simulink model "Deployment_Env"  (R2024a)
settings: Solver=ode1  StartTime=0.0  StopTime=inf  FixedStep=0.002  RelTol=1e-3  EnableMultiTasking=on
PostLoadFcn:
  | qc_set_target_type(getConfigSet(bdroot, 'QUARC Default Target Configuration'));
undefined symbols (not defined in the file or in its folder): HIL, Lp, qc_get_step_size
libraries: quarc_library x9, simulink x3, simulink_extras x2, rllib x1
settings Model: SimulationMode=external  ExtModeTrigDuration=5000  Creator=pmartin  LastModifiedBy=sameb
settings SolverCC: AlgebraicLoopSolver=TrustRegion  PositivePriorityOrder=on  AutoInsertRateTranBlk=on
settings DataIOCC: LimitDataPoints=on  SaveFormat=Array  SignalLoggingSaveFormat=ModelDataLogs  ReturnWorkspaceOutputs=off
settings OptimizationCC: ExpressionDepthLimit=2147483647  InitFltsAndDblsToZero=on
settings DebuggingCC: SaveWithParameterizedLinksMsg=none  UnderspecifiedInitializationDetection=Classic  MergeDetectMultiDrivingBlocksExec=none  SolverPrmCheckMsg=warning  MultiTaskDSMMsg=warning  MultiTaskCondExecSysMsg=none  FcnCallInpInsideContextMsg=warning  UnconnectedInputMsg=warning  UnconnectedOutputMsg=warning  UnconnectedLineMsg=warning  StateNameClashWarn=warning  SFUnexpectedBacktrackingDiag=warning  SFNoUnconditionalDefaultTransitionDiag=warning  SFExecutionAtInitializationDiag=none  ArithmeticOperatorsInVariantConditions=warning
settings HardwareCC: ProdBitPerPointer=32  ProdBitPerSizeT=32  ProdBitPerPtrDiffT=32  ProdLargestAtomicFloat=None  ProdIntDivRoundTo=Undefined  ProdEndianess=Unspecified  ProdWordSize=32  ProdHWDeviceType=32-bit Generic
settings ModelReferenceCC: EnableRefExpFcnMdlSchedulingChecks=on  PropagateSignalLabelsOutOfModel=off
settings SFSimCC: SimUseLocalCustomCode=off  CustomCodeUndefinedFunction=UseInterfaceOnly
settings RTWCC: Description=QUARC Win64 Target  SystemTargetFile=quarc_win64.tlc  TemplateMakefile=quarc_default_tmf  RTWUseLocalCustomCode=off  GPUComputeCapability=3.5  DLArmComputeVersion=19.05
settings CodeAppCC: StateflowObjectComments=on
settings STFCustomTargetCC: TargetPreCompLibLocation=C:\PROGRA~3\QUARC\lib\2020b\win64\release  TargetLangStandard=C89/C90 (ANSI)  ConcurrentExecutionCompliant=on  UseToolchainInfoCompliant=off  SystemTargetFile=quarc_win64.tlc
settings GRTTargetCC: TargetPreCompLibLocation=C:\PROGRA~3\QUARC\lib\2020b\win64\release  TargetLangStandard=C89/C90 (ANSI)  ParMdlRefBuildCompliant=off  CompOptLevelCompliant=off  CombineOutputUpdateFcns=off  MatFileLogging=off  CPPClassGenCompliant=off  GRTInterface=on  UseToolchainInfoCompliant=off  ExtMode=on  ExtModeMexFile=quarc_comm
settings ConfigComp: CovMetricSettings=dw  CovSaveCumulativeToWorkspaceVar=on  CovSaveSingleToWorkspaceVar=on  CovExternalEMLEnable=off

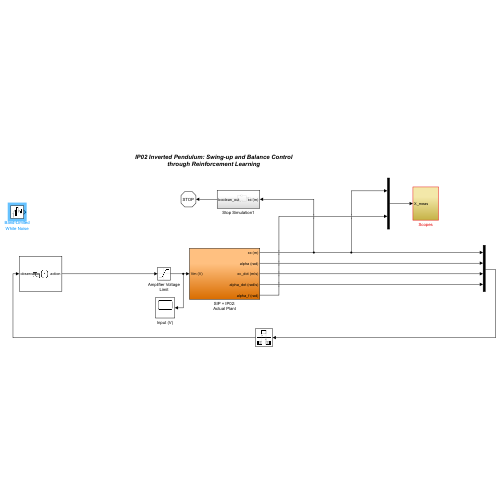
[thumbnail: Simulink's stored preview of the top-level diagram]
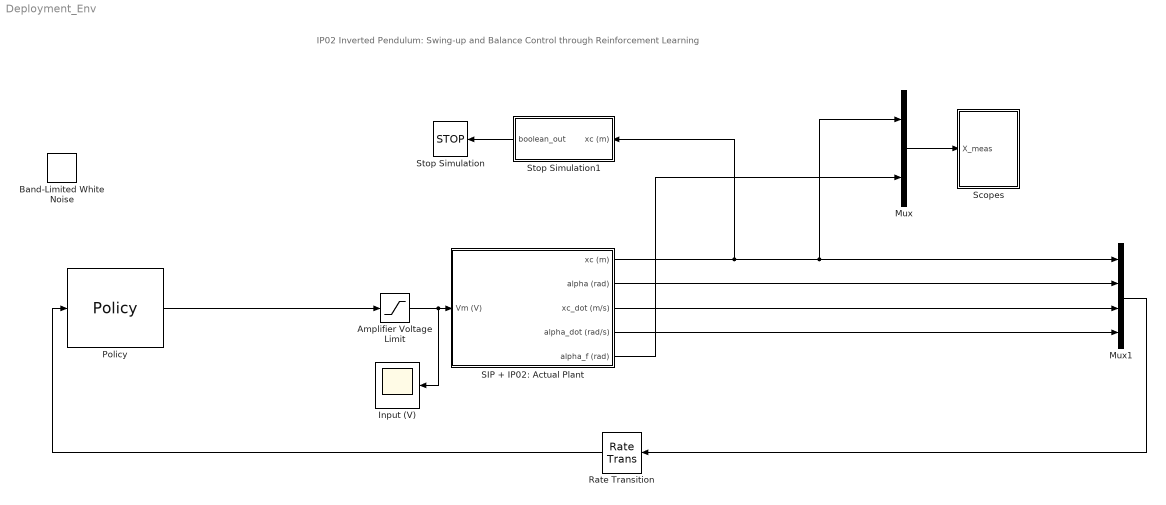
== system Deployment_Env ==
  note: IP02 Inverted Pendulum: Swing-up and Balance Control through Reinforcement Learning
  Amplifier Voltage Limit : Saturate  UpperLimit=10  LowerLimit=-10
  Band-Limited White Noise : simulink/Sources/Band-Limited White Noise  Cov=[0.1]  Ts=0.1  seed=[23341]
  Input (V) : Scope
  Mux : Mux  Inputs=2
  Mux1 : Mux
  Policy : rllib/Policy  MATFile=blockAgentData.mat  PolicyParamsAsInput=off  PolicyParamsBusName=policy_param_bus  SimUsingCodegen=off
  Rate Transition : RateTransition  OutPortSampleTime=0.05
  SIP + IP02: Actual Plant : Subsystem
  Scopes : Subsystem
  Stop Simulation : Stop
  Stop Simulation1 : Subsystem
  wires:
  Amplifier Voltage Limit/1 -> Input (V)/1, SIP + IP02: Actual Plant/1(Vm (V))
  SIP + IP02: Actual Plant/1(xc (m)) -> Stop Simulation1/1(xc (m)), Mux/1, Mux1/1
  Mux/1 -> Scopes/1(X_meas)
  SIP + IP02: Actual Plant/2(alpha (rad)) -> Mux1/2
  SIP + IP02: Actual Plant/5(alpha_f (rad)) -> Mux/2
  SIP + IP02: Actual Plant/3(xc_dot (m/s)) -> Mux1/3
  SIP + IP02: Actual Plant/4(alpha_dot (rad/s)) -> Mux1/4
  Policy/1 -> Amplifier Voltage Limit/1
  Mux1/1 -> Rate Transition/1
  Rate Transition/1 -> Policy/1
  Stop Simulation1/1(boolean_out) -> Stop Simulation/1

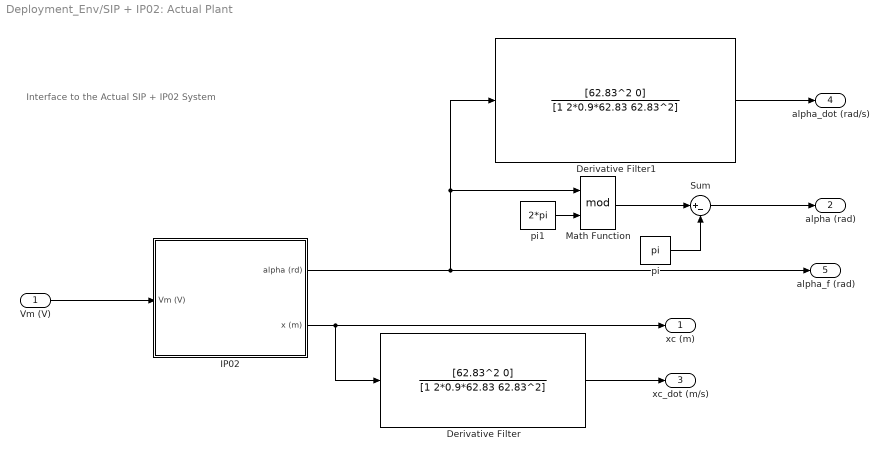
== system Deployment_Env/SIP + IP02: Actual Plant ==
  note: Interface to the Actual
      | SIP + IP02 System
  Vm (V) : Inport
  Derivative Filter : TransferFcn  Numerator=[62.83^2 0]  Denominator=[1 2*0.9*62.83 62.83^2]
  Derivative Filter1 : TransferFcn  Numerator=[62.83^2 0]  Denominator=[1 2*0.9*62.83 62.83^2]
  "IP02 " : Subsystem
  Math Function : Math  Operator=mod  SignedPower=on
  Sum : Sum  Inputs=|+-  InputSameDT=on  SaturateOnIntegerOverflow=on  OutDataTypeStr=Inherit: Same as first input
  pi : Constant  Value=pi
  pi1 : Constant  Value=2*pi
  xc (m) : Outport  InitialOutput=0
  alpha (rad) : Outport  Port=2  InitialOutput=0
  xc_dot (m/s) : Outport  Port=3  InitialOutput=0
  alpha_dot (rad/s) : Outport  Port=4  InitialOutput=0
  alpha_f (rad) : Outport  Port=5  InitialOutput=0
  wires:
  "IP02 "/2(x (m)) -> xc (m)/1, Derivative Filter/1
  Derivative Filter1/1 -> alpha_dot (rad/s)/1
  Derivative Filter/1 -> xc_dot (m/s)/1
  pi1/1 -> Math Function/2
  pi/1 -> Sum/2
  Sum/1 -> alpha (rad)/1
  Math Function/1 -> Sum/1
  Vm (V)/1 -> "IP02 "/1(Vm (V))
  "IP02 "/1(alpha (rd)) -> Math Function/1, Derivative Filter1/1, alpha_f (rad)/1

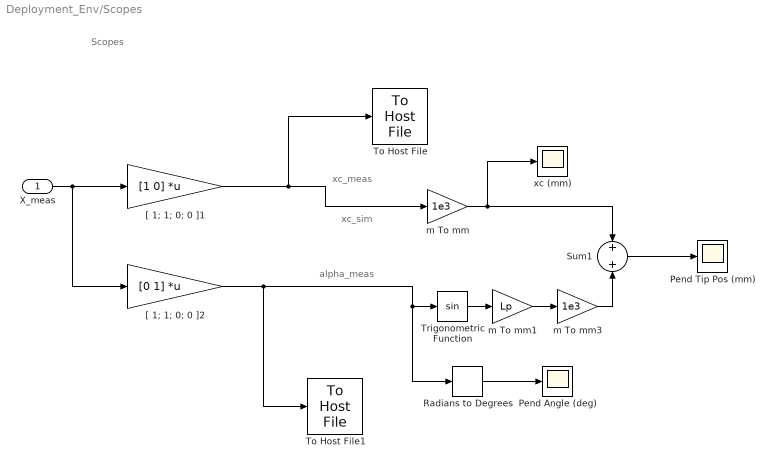
== system Deployment_Env/Scopes ==
  note: xc_meas
  note: alpha_meas
  note: xc_sim
  note: Scopes
  X_meas : Inport
  Pend Angle (deg) : Scope
  Pend Tip Pos (mm) : Scope
  Radians to Degrees : simulink_extras/Transformations/Radians to Degrees
  Sum1 : Sum  Inputs=+|+  InputSameDT=on  SaturateOnIntegerOverflow=on  OutDataTypeStr=Inherit: Same as first input
  To Host File : quarc_library/Sinks/To Host/To Host File  file_name=x_meas.mat  variable_name=x_meas  decimation=1  sample_time=0.01  file_format=MAT-file v.4  options=No header or footer  append=off  final_file_name=x_meas.mat  bitrate=2000000
  To Host File1 : quarc_library/Sinks/To Host/To Host File  file_name=alpha_meas.mat  variable_name=alpha_meas  decimation=1  sample_time=0.01  file_format=MAT-file v.4  options=No header or footer  append=off  final_file_name=alpha_meas.mat  bitrate=2000000
  Trigonometric Function : Trigonometry
  "[ 1; 1; 0; 0 ]1" : Gain  Gain=[1 0]  Multiplication=Matrix(K*u)  SaturateOnIntegerOverflow=on  OutDataTypeStr=Inherit: Same as input  ParamDataTypeStr=Inherit: Same as input
  "[ 1; 1; 0; 0 ]2" : Gain  Gain=[0 1]  Multiplication=Matrix(K*u)  SaturateOnIntegerOverflow=on  OutDataTypeStr=Inherit: Same as input  ParamDataTypeStr=Inherit: Same as input
  m To mm : Gain  Gain=1e3  SaturateOnIntegerOverflow=on  OutDataTypeStr=Inherit: Same as input  ParamDataTypeStr=Inherit: Same as input
  m To mm1 : Gain  Gain=Lp  SaturateOnIntegerOverflow=on  OutDataTypeStr=Inherit: Same as input  ParamDataTypeStr=Inherit: Same as input
  m To mm3 : Gain  Gain=1e3  SaturateOnIntegerOverflow=on  OutDataTypeStr=Inherit: Same as input  ParamDataTypeStr=Inherit: Same as input
  xc (mm) : Scope
  wires:
  m To mm/1 -> Sum1/1, xc (mm)/1
  X_meas/1 -> "[ 1; 1; 0; 0 ]1"/1, "[ 1; 1; 0; 0 ]2"/1
  m To mm1/1 -> m To mm3/1
  Trigonometric Function/1 -> m To mm1/1
  m To mm3/1 -> Sum1/2
  Sum1/1 -> Pend Tip Pos (mm)/1
  Radians to Degrees/1 -> Pend Angle (deg)/1
  "[ 1; 1; 0; 0 ]1"/1 -> To Host File/1, m To mm/1
  "[ 1; 1; 0; 0 ]2"/1 -> To Host File1/1, Trigonometric Function/1, Radians to Degrees/1

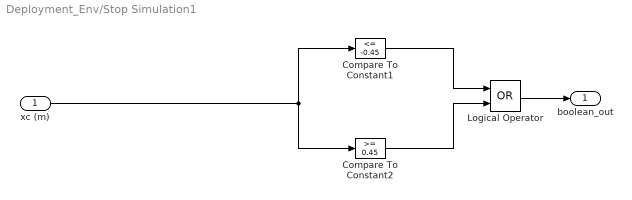
== system Deployment_Env/Stop Simulation1 ==
  xc (m) : Inport
  Compare To Constant1 : simulink/Logic and Bit Operations/Compare To Constant  relop=<=  const=-0.45  OutDataTypeStr=boolean
  Compare To Constant2 : simulink/Logic and Bit Operations/Compare To Constant  relop=>=  const=0.45  OutDataTypeStr=boolean
  Logical Operator : Logic  Operator=OR  AllPortsSameDT=off  OutDataTypeStr=boolean
  boolean_out : Outport
  wires:
  Logical Operator/1 -> boolean_out/1
  Compare To Constant2/1 -> Logical Operator/2
  Compare To Constant1/1 -> Logical Operator/1
  xc (m)/1 -> Compare To Constant1/1, Compare To Constant2/1

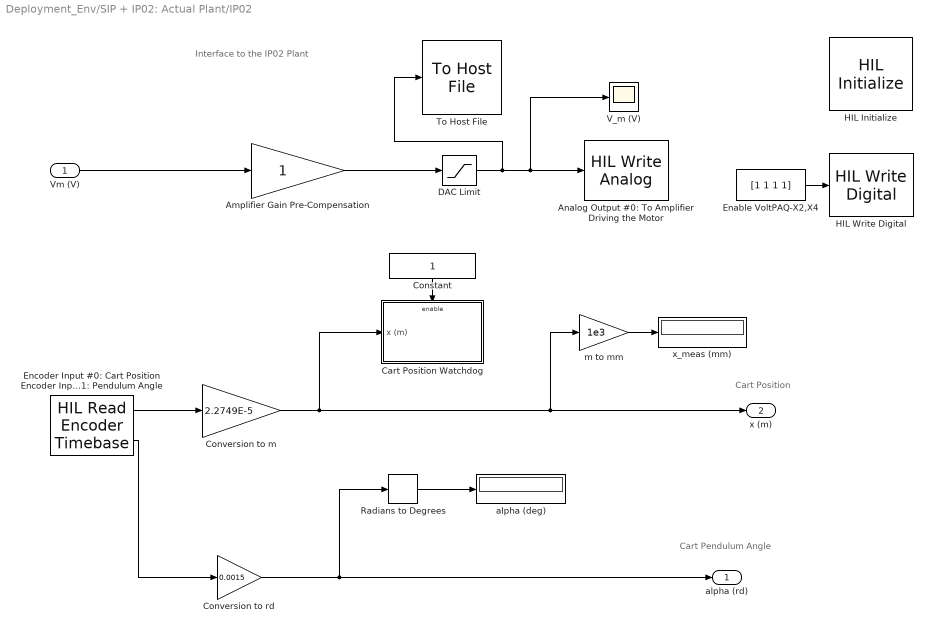
== system Deployment_Env/SIP + IP02: Actual Plant/IP02  ==
  note: Cart Pendulum Angle
  note: Cart Position
  note: Interface to the IP02 Plant
  Vm (V) : Inport
  Amplifier Gain Pre-Compensation : Gain  SaturateOnIntegerOverflow=on  OutDataTypeStr=Inherit: Same as input  ParamDataTypeStr=Inherit: Same as input
  Analog Output #0: To Amplifier Driving the Motor : quarc_library/Data Acquisition/Generic/Immediate I//O/HIL Write Analog  Tag=unassigned  object_name=HIL-1  channels=0  sample_time=-1  active=on  vector_input=on
  Cart Position Watchdog : Subsystem  TreatAsAtomicUnit=on
  Constant : Constant
  Conversion to m : Gain  Gain=2.2749E-5  SaturateOnIntegerOverflow=on  OutDataTypeStr=Inherit: Same as input  ParamDataTypeStr=Inherit: Same as input
  Conversion to rd : Gain  Gain=0.0015  SaturateOnIntegerOverflow=on  OutDataTypeStr=Inherit: Same as input  ParamDataTypeStr=Inherit: Same as input
  DAC Limit : Saturate  UpperLimit=10  LowerLimit=-10
  Enable VoltPAQ-X2,X4 : Constant  Value=[1 1 1 1]
  Encoder Input #0: Cart Position Encoder Input #1: Pendulum Angle : quarc_library/Data Acquisition/Generic/Timebases/HIL Read Encoder Timebase  Tag=unassigned  object_name=HIL-1  clock=0  channels=[0 1]  active=on  vector_output=off  data_type_mode=Inherit via back propagation  data_type=double  overflow_mode=Error on overflow  samples_in_buffer=max(ceil(1/qc_get_step_size), 1)
  HIL Initialize : quarc_library/Data Acquisition/Generic/Configuration/HIL Initialize  object_name=HIL-1  board_type=q2_usb  board_number=0  board_options=d0=digital;d1=digital;led=auto;update_rate=normal  exclusive=off  active=off  hardware_clocks=[0:2]  clock_modes=[]  initial_clock_frequencies=[]  set_clock_params_at_start=off  set_clock_params_at_switch_in=off  set_clock_frequencies_at_start=off  set_clock_frequencies_at_switch_in=off  analog_input_channels=[0:1]  analog_input_configurations=[]  analog_input_maximums=10  analog_input_minimums=-10  set_analog_input_params_at_start=on  set_analog_input_params_at_switch_in=off  analog_output_channels=[0:1]  analog_output_maximums=10  analog_output_minimums=-10  initial_analog_outputs=[0]  final_analog_outputs=[0]  watchdog_analog_outputs=0  set_analog_output_params_at_start=on  set_analog_output_params_at_switch_in=off  set_analog_outputs_at_start=on  set_analog_outputs_at_switch_in=off  set_analog_outputs_at_terminate=on  set_analog_outputs_at_switch_out=off  set_analog_outputs_on_watchdog=off  digital_input_channels=[]  digital_output_channels=[0:7]  digital_output_configuration=[]  initial_digital_outputs=[0]  final_digital_outputs=[0]  watchdog_digital_outputs=[0]  set_digital_output_params_at_start=off  set_digital_output_params_at_switch_in=off  set_digital_outputs_at_start=on  set_digital_outputs_at_switch_in=off  set_digital_outputs_at_terminate=on  set_digital_outputs_at_switch_out=off  set_digital_outputs_on_watchdog=off  encoder_channels=[0:1]  quadrature=[4]  encoder_filter_frequency=[]  initial_encoder_counts=[0]  set_encoder_params_at_start=on  set_encoder_params_at_switch_in=off  set_encoder_counts_at_start=on  set_encoder_counts_at_switch_in=off  pwm_channels=[]  pwm_modes=[0]  pwm_frequency=1/0.020  pwm_configuration=[]  pwm_alignment=[]  pwm_polarity=[]  pwm_leading_deadband=[]  pwm_trailing_deadband=[]  initial_pwm_outputs=[0]  final_pwm_outputs=[0]  watchdog_pwm_outputs=[0]  set_pwm_params_at_start=on  set_pwm_params_at_switch_in=off  set_pwm_outputs_at_start=on  set_pwm_outputs_at_switch_in=off  set_pwm_outputs_at_terminate=on  set_pwm_outputs_at_switch_out=off  set_pwm_outputs_on_watchdog=off  other_output_channels=[]  initial_other_outputs=[]  final_other_outputs=[]  watchdog_other_outputs=[]  set_other_outputs_at_start=off  set_other_outputs_at_switch_in=off  set_other_outputs_at_terminate=off  set_other_outputs_at_switch_out=off  set_other_outputs_on_watchdog=off
  HIL Write Digital : quarc_library/Data Acquisition/Generic/Immediate I//O/HIL Write Digital  object_name=HIL-1  channels=[0:3]  sample_time=-1  active=off  vector_input=on
  Radians to Degrees : simulink_extras/Transformations/Radians to Degrees
  To Host File : quarc_library/Sinks/To Host/To Host File  file_name=input.mat  variable_name=input  decimation=1  sample_time=0.01  file_format=MAT-file v.4  options=No header or footer  append=off  final_file_name=input.mat  bitrate=2000000
  V_m (V) : Scope
  alpha (deg) : Display
      settings: Decimation=100
  m to mm : Gain  Gain=1e3  SaturateOnIntegerOverflow=on  OutDataTypeStr=Inherit: Same as input  ParamDataTypeStr=Inherit: Same as input
  x_meas (mm) : Display
      settings: Decimation=100
  alpha (rd) : Outport  InitialOutput=0
  x (m) : Outport  Port=2  InitialOutput=0
  wires:
  Encoder Input #0: Cart Position Encoder Input #1: Pendulum Angle/1 -> Conversion to m/1
  Conversion to m/1 -> Cart Position Watchdog/1(x (m)), x (m)/1, m to mm/1
  Amplifier Gain Pre-Compensation/1 -> DAC Limit/1
  m to mm/1 -> x_meas (mm)/1
  Encoder Input #0: Cart Position Encoder Input #1: Pendulum Angle/2 -> Conversion to rd/1
  Radians to Degrees/1 -> alpha (deg)/1
  Conversion to rd/1 -> Radians to Degrees/1, alpha (rd)/1
  Constant/1 -> Cart Position Watchdog/Enable
  Vm (V)/1 -> Amplifier Gain Pre-Compensation/1
  Enable VoltPAQ-X2,X4/1 -> HIL Write Digital/1
  DAC Limit/1 -> To Host File/1, Analog Output #0: To Amplifier Driving the Motor/1, V_m (V)/1

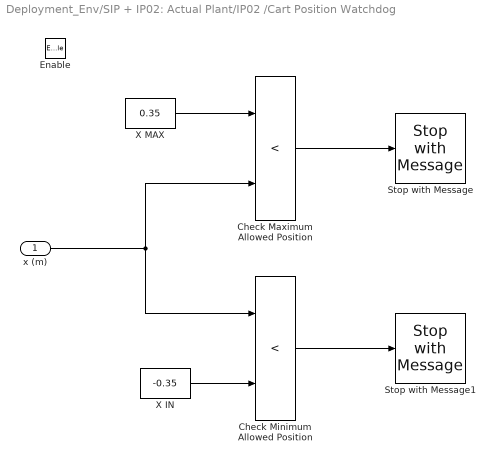
== system Deployment_Env/SIP + IP02: Actual Plant/IP02 /Cart Position Watchdog ==
  x (m) : Inport
  Enable : EnablePort
  Check Maximum Allowed Position : RelationalOperator  Operator=<
  Check Minimum Allowed Position : RelationalOperator  Operator=<
  Stop with Message : quarc_library/Sinks/Error Handling/Stop with Message  message_type=Fixed error message  message_icon=Error  message=Maximum Limit Reached.
  Stop with Message1 : quarc_library/Sinks/Error Handling/Stop with Message  message_type=Fixed error message  message_icon=Error  message=Minimum Limit Reached.
  X IN : Constant  Value=-0.35
  X MAX : Constant  Value=0.35
  wires:
  Check Maximum Allowed Position/1 -> Stop with Message/1
  x (m)/1 -> Check Minimum Allowed Position/1, Check Maximum Allowed Position/2
  X IN/1 -> Check Minimum Allowed Position/2
  Check Minimum Allowed Position/1 -> Stop with Message1/1
  X MAX/1 -> Check Maximum Allowed Position/1
